simulink model "trirtyseven"  (R2022b)
settings: Solver=VariableStepAuto  StartTime=0.0  StopTime=10.0  RelTol=1e-3
values from neighbouring files (symbols this model uses):
  A = [0, 1; g/L, -gamma/(M*L)]    [pendulum.m]
  B = [0; 1]    [pendulum.m]
  K = inv(R) * B' * P    [pendulum.m]
  x0 = [pi; 1]    [pendulum.m]
settings Model: Creator=User  LastModifiedBy=User

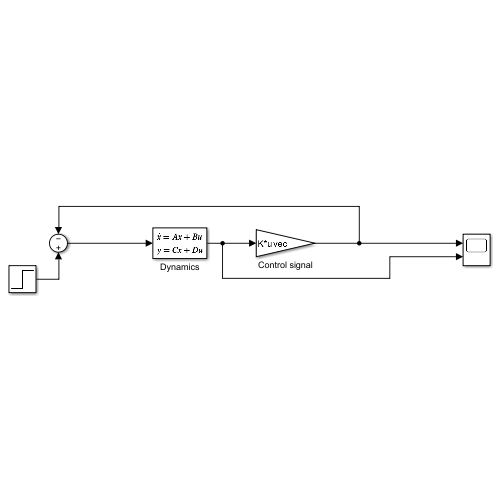
[thumbnail: Simulink's stored preview of the top-level diagram]
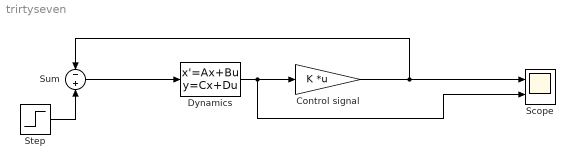
== system trirtyseven ==
  Control signal : Gain  Gain=K  Multiplication=Matrix(K*u) (u vector)
  Dynamics : StateSpace  A=A  B=B  C=eye(2)  D=[0; 0]  InitialCondition=x0  ContinuousStateAttributes='position'
  Scope : Scope  NumInputPorts=2
  Step : Step  After=3  SampleTime=0
  Sum : Sum  Inputs=-|+
  wires:
  Control signal/1 -> Sum/1, Scope/1
  Step/1 -> Sum/2
  Sum/1 -> Dynamics/1
  Dynamics/1 -> Control signal/1, Scope/2
